simulink model "ob_reg"  (R2016b)
settings: Solver=FixedStepAuto  StartTime=0.0  StopTime=15  FixedStep=0.01  RelTol=1e-3
values from neighbouring files (symbols this model uses):
  A = [2  -4  -1; 4  -2  -1; -4  0  -1]    [matlab.mat]    (also in obserwator_stanu.m = [2 -4 -1)
  B = [0 0 -2]    [matlab.mat]    (also in obserwator_stanu.m = [0;0;-2])
  C = [1 0 0]    [matlab.mat]    (also in obserwator_stanu.m)
  D = 0    [matlab.mat]    (also in obserwator_stanu.m = [0])
  H = [11 -3.54166666667 12.9166666667]    [matlab.mat]    (also in obserwator_stanu.m = L')
undefined symbols (not defined in the file or in its folder): sigbuilder_block
settings Model: Creator=lenovo  LastModifiedBy=lenovo

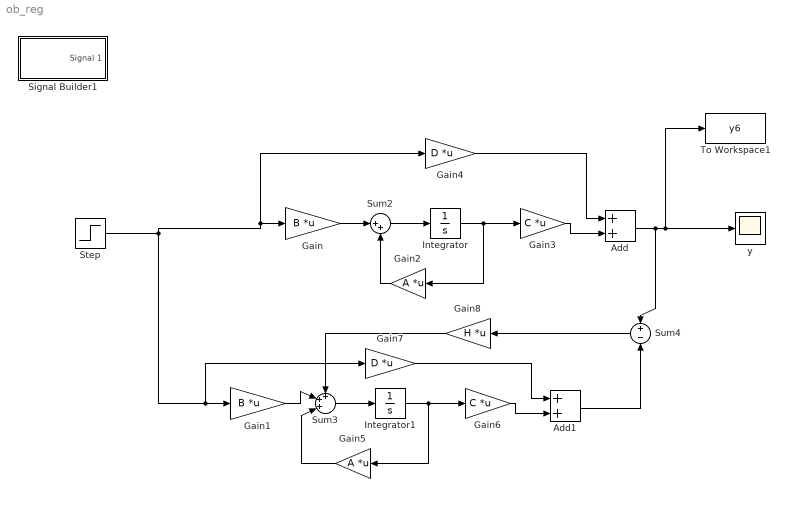
== system ob_reg ==
  Add : Sum
  Add1 : Sum
  Gain : Gain  Gain=B  Multiplication=Matrix(K*u)
  Gain1 : Gain  Gain=B  Multiplication=Matrix(K*u)
  Gain2 : Gain  Gain=A  Multiplication=Matrix(K*u)
  Gain3 : Gain  Gain=C  Multiplication=Matrix(K*u)
  Gain4 : Gain  Gain=D  Multiplication=Matrix(K*u)
  Gain5 : Gain  Gain=A  Multiplication=Matrix(K*u)
  Gain6 : Gain  Gain=C  Multiplication=Matrix(K*u)
  Gain7 : Gain  Gain=D  Multiplication=Matrix(K*u)
  Gain8 : Gain  Gain=H  Multiplication=Matrix(K*u)
  Integrator : Integrator
  Integrator1 : Integrator
  Signal Builder1 : Subsystem  Tag=STV Subsys  LoadFcn=sigbuilder_block('load');  StartFcn=sigbuilder_block('start');  StopFcn=sigbuilder_block('stop');  ClipboardFcn=sigbuilder_block('clipboard');  mask(Sigbuilder block){tuvar=[0:10]}
      mask help: Simulink:masks:SigbuilderBlock_MD
      mask init:
      | if ~strcmp(get_param(bdroot(gcbh),'SimulationStatus'),'stopped') tuvar = sigbuilder_block('maskInit'); end
      settings: CopyFcn=sigbuilder_block('copy');  DeleteFcn=sigbuilder_block('delete');  ModelCloseFcn=sigbuilder_block('modelClose');  PreSaveFcn=sigbuilder_block('preSave');  PauseFcn=sigbuilder_block('pause');  ContinueFcn=sigbuilder_block('continue');  NameChangeFcn=sigbuilder_block('namechange');  OpenFcn=sigbuilder_block('open',[437.25 153.75 550.5 359.25 ]);  CloseFcn=sigbuilder_block('close');
      mask Display: plot(0, 0, 100, 100,[2, 2, 32, 32, 2], [68, 8, 8, 68, 68],[32, 2], [38, 38], [32, 19, 2],[53, 60, 44], [32, 17, 17, 2],[16, 16, 31, 31]);txt = getActiveGroup(gcbh);text(2, 100, txt,'verticalAlignment', 'top');
  Step : Step  Time=0  SampleTime=0
  Sum2 : Sum  Inputs=|++
  Sum3 : Sum  Inputs=+++|
  Sum4 : Sum  Inputs=+|-
  To Workspace1 : ToWorkspace  VariableName=y6  SaveFormat=Timeseries  SampleTime=-1
  y : Scope
  wires:
  Add/1 -> Sum4/1, To Workspace1/1, y/1
  Gain2/1 -> Sum2/2
  Gain/1 -> Sum2/1
  Sum2/1 -> Integrator/1
  Integrator/1 -> Gain2/1, Gain3/1
  Gain3/1 -> Add/2
  Gain4/1 -> Add/1
  Step/1 -> Gain4/1, Gain/1, Gain7/1, Gain1/1
  Sum3/1 -> Integrator1/1
  Integrator1/1 -> Gain5/1, Gain6/1
  Gain6/1 -> Add1/2
  Gain7/1 -> Add1/1
  Add1/1 -> Sum4/2
  Gain1/1 -> Sum3/2
  Gain5/1 -> Sum3/3
  Sum4/1 -> Gain8/1
  Gain8/1 -> Sum3/1

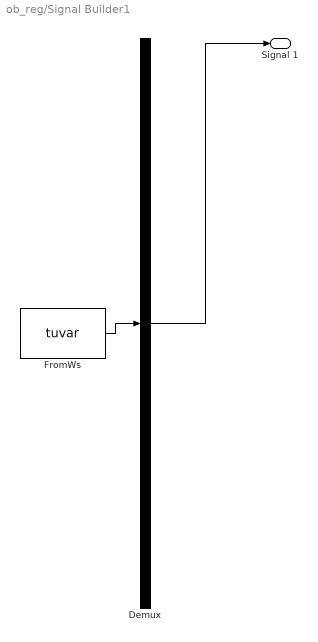
== system ob_reg/Signal Builder1 ==
  Demux : Demux  Tag=STV Demux  Outputs=1
  FromWs : FromWorkspace  Tag=STV FromWs  VariableName=tuvar  SampleTime=0
      SigBuilderData=|
      | common.afterFinalStr = 'Extrapolate'
      | common.sampleTime = 0
      | dataSet.timeRange = [0 10]
      | dataSet.name = 'Group 1'
      | sbobj.Groups.Name = 'Group 1'
      | sbobj.Groups.Signals.Name = 'Signal 1'
      | sbobj.Groups.Signals.XData = [0 7.22 7.22 7.46 7.46 10]
      | sbobj.Groups.Signals.YData = [0 0 1.005 1.005 0 0]
  Signal 1 : Outport  Tag=STV Outport
  wires:
  Demux/1 -> Signal 1/1
  FromWs/1 -> Demux/1
